simulink model "GPCA_AlarmDebug1"  (Simulink 9.0)
settings: Solver=FixedStepDiscrete  StartTime=0.0  StopTime=19.8  FixedStep=0.200000  RelTol=1e-3  EnableMultiTasking=on
model workspace (MAT data in the model file):
  already_pp = 1
  input_struct.time = [0; 0.2; 0.4; 0.6; 0.8; 1; 1.2; 1.4; 1.6; 1.8; 2; 2.2; 2.4; 2.6; 2.8; 3; 3.2; 3.4; 3.6; 3.8; 4; 4.2; 4.4; 4.6; 4.8; 5; 5.2; 5.4; 5.6; 5.8; 6; 6.2; 6.4; 6.6; 6.8; 7; 7.2; 7.4; 7.6; 7.8; 8; 8.2; 8.4; 8.6; 8.8; 9; 9.2; 9.4; 9.6; 9.8; 10; 10.2; 10.4; 10.6; 10.8; 11; 11.2; 11.4; 11.6; 11.8; 12; 12.2; 12.4; 12.6; 12.8; 13; 13.2; 13.4; 13.6; 13.8; 14; 14.2; 14.4; 14.6; 14.8; 15; 15.2; 15.4; 15.6; 15.8; 16; 16.2; 16.4; 16.6; 16.8; 17; 17.2; 17.4; 17.6; 17.8; 18; 18.2; 18.4; 18.6; 18.8; 19; 19.2; 19.4; 19.6; 19.8]
  input_struct.signals(1).name = 'c1'
  input_struct.signals(1).values = [1; 1; 0; 1; 1; 0; 0; 1; 1; 1; 0; 1; 1; 0; 1; 0; 0; 1; 1; 1; 1; 0; 1; 1; 1; 1; 1; 0; 1; 0; 1; 0; 0; 0; 0; 1; 1; 0; 1; 0; 0; 0; 1; 1; 0; 0; 0; 1; 1; 1; 0; 1; 1; 0; 0; 0; 1; 0; 1; 0; 1; 0; 1; 1; 1; 1; 1; 0; 0; 0; 1; 0; 1; 0; 1; 0; 0; 0; 1; 0; 0; 1; 1; 1; 1; 0; 1; 1; 0; 1; 0; 0; 1; 1; 1; 0; 1; 0; 0; 0]
  input_struct.signals(1).dimensions = 1
  input_struct.signals(2).name = 'c2'
  input_struct.signals(2).values = [0; 1; 0; 1; 0; 1; 0; 1; 1; 1; 0; 0; 0; 1; 0; 1; 1; 1; 0; 0; 0; 1; 0; 1; 1; 1; 0; 0; 0; 1; 0; 1; 0; 0; 0; 0; 1; 1; 1; 0; 1; 1; 0; 1; 0; 0; 0; 0; 0; 0; 0; 0; 1; 1; 0; 0; 0; 1; 0; 0; 1; 0; 0; 0; 0; 0; 1; 1; 1; 0; 0; 0; 1; 0; 0; 0; 1; 1; 1; 0; 1; 0; 1; 0; 1; 0; 0; 1; 1; 0; 1; 1; 0; 0; 0; 0; 1; 1; 1; 1]
  input_struct.signals(2).dimensions = 1
  input_struct.signals(3).name = 'c3'
  input_struct.signals(3).values = [1; 0; 1; 1; 0; 1; 1; 1; 1; 1; 0; 0; 0; 0; 1; 0; 0; 0; 0; 0; 0; 1; 0; 0; 1; 1; 0; 0; 0; 0; 1; 0; 1; 1; 0; 0; 0; 0; 0; 1; 0; 0; 1; 0; 1; 1; 0; 1; 0; 0; 1; 1; 1; 0; 0; 1; 1; 0; 0; 1; 0; 1; 1; 1; 0; 0; 0; 1; 0; 1; 0; 1; 0; 1; 1; 1; 1; 0; 1; 0; 0; 1; 0; 0; 1; 1; 1; 1; 1; 1; 0; 0; 1; 0; 0; 0; 1; 1; 0; 0]
  input_struct.signals(3).dimensions : numeric (value not decoded)
settings Model: SuppressorTable=22 serialization::archive 11 0 6 0 0 0 0 0  Creator=bourbouh  LastModifiedBy=hbourbou
settings DataIOCC: ExternalInput=input_struct  LoadExternalInput=on  SaveFormat=Structure  SaveState=on
settings DebuggingCC: AlgebraicLoopMsg=error  ArtificialAlgebraicLoopMsg=error  UnderspecifiedInitializationDetection=Simplified  MergeDetectMultiDrivingBlocksExec=error  SingleTaskRateTransMsg=error
settings HardwareCC: ProdBitPerPointer=64  ProdBitPerSizeT=64  ProdBitPerPtrDiffT=64  ProdLargestAtomicFloat=Float  ProdIntDivRoundTo=Zero  ProdEndianess=LittleEndian  ProdWordSize=64  ProdHWDeviceType=Intel->x86-64 (Windows64)
settings ModelReferenceCC: PropagateSignalLabelsOutOfModel=on
settings GRTTargetCC: GeneratePreprocessorConditionals=Disable all  ExtMode=on

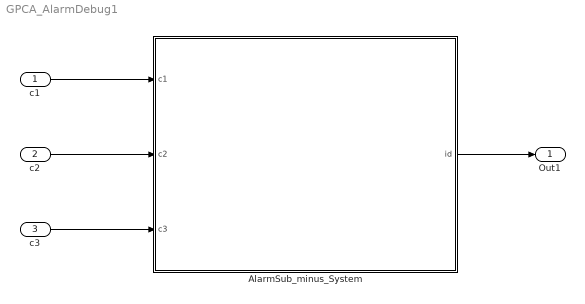
== system GPCA_AlarmDebug1 ==
  c1 : Inport  OutDataTypeStr=boolean  PortDimensions=1
  c2 : Inport  Port=2  OutDataTypeStr=boolean  PortDimensions=1
  c3 : Inport  Port=3  OutDataTypeStr=boolean  PortDimensions=1
  AlarmSub_minus_System : Stateflow chart  TreatAsAtomicUnit=on
  Out1 : Outport
  wires:
  AlarmSub_minus_System/1(id) -> Out1/1
  c3/1 -> AlarmSub_minus_System/3(c3)
  c2/1 -> AlarmSub_minus_System/2(c2)
  c1/1 -> AlarmSub_minus_System/1(c1)

== stateflow chart AlarmSub_minus_System ==
  state Alarms
    state Notification1 [parallel]
      en: id = 21;
      settings: executionOrder=1
      state A
        en : id = 3;
      state B
        en : id = 4;
      (default) -> A
      Alarms.Notification1.B -> A : [c1]
      A -> Alarms.Notification1.B : [c2]
    state Notification2 [parallel]
      en: id = 22;
      settings: executionOrder=2
      state B
        en : id = 5;
  state NOT_ON
    en: id = 1;
  (default) -> Alarms [order 1] : [c1]
  (default) -> NOT_ON [order 2]
  NOT_ON -> Alarms : [c2]
  Alarms -> NOT_ON : [c3]
  data: id output double; c1 input boolean; c2 input boolean; c3 input boolean
